simulink model "Diff_Amp"  (Simulink 8.9)
settings: Solver=ode15s  StartTime=0.0  StopTime=0.2  MaxStep=0.00002  RelTol=1e-3  EnableMultiTasking=on
libraries: fl_lib x9, nesl_utility x2
settings Model: Creator=subramanian.krishnan  LastModifiedBy=hac
settings OptimizationCC: ExpressionDepthLimit=2147483647  InitFltsAndDblsToZero=on

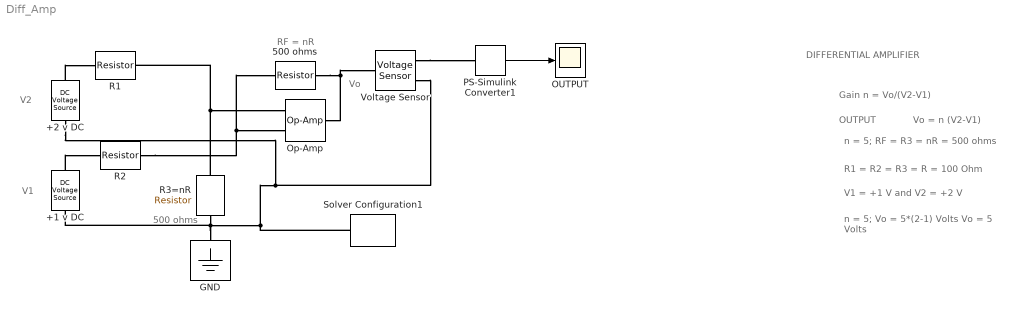
== system Diff_Amp ==
  note: DIFFERENTIAL AMPLIFIER
  note: V2
  note: V1
  note: Vo
  note: Vo = n (V2-V1)
  note: n = 5; Vo = 5*(2-1) Volts
      | Vo = 5 Volts
  note: OUTPUT
  note: RF = nR
  note: R1 = R2 = R3 = R = 100 Ohm
  note: V1 = +1 V and V2 = +2 V
  note: Gain n = Vo/(V2-V1)
  note: 500 ohms
  note: n = 5; RF = R3 = nR = 500 ohms
  +1 v DC : fl_lib/Electrical/Electrical Sources/DC Voltage Source  v0=1 V
  "+2 v DC " : fl_lib/Electrical/Electrical Sources/DC Voltage Source  v0=2 V
  500 ohms : fl_lib/Electrical/Electrical Elements/Resistor  R=500 Ohm  i_specify=off  i_priority=None  i=0 A  i_nominal_specify=off  i_nominal_unit=A  i_nominal_value=1  v_specify=off  v_priority=None  v=0 V  v_nominal_specify=off  v_nominal_unit=V  v_nominal_value=1
  GND : fl_lib/Electrical/Electrical Elements/Electrical Reference
  OUTPUT : Scope
  Op-Amp : fl_lib/Electrical/Electrical Elements/Op-Amp  outI_specify=off  outI_priority=None  outI=0 A  outI_nominal_specify=off  outI_nominal_unit=A  outI_nominal_value=1
  PS-Simulink Converter1 : nesl_utility/PS-Simulink Converter  PhysicalDomain=network_engine_domain  SubClassName=ps_output  LeftPortType=input  RightPortType=output  PseudoPeriodic=off  Frequencies=[]  Unit=1  AffineConversion=off
  R1 : fl_lib/Electrical/Electrical Elements/Resistor  R=100 Ohm  i_specify=off  i_priority=None  i=0 A  i_nominal_specify=off  i_nominal_unit=A  i_nominal_value=1  v_specify=off  v_priority=None  v=0 V  v_nominal_specify=off  v_nominal_unit=V  v_nominal_value=1
  R2 : fl_lib/Electrical/Electrical Elements/Resistor  R=100 Ohm  i_specify=off  i_priority=None  i=0 A  i_nominal_specify=off  i_nominal_unit=A  i_nominal_value=1  v_specify=off  v_priority=None  v=0 V  v_nominal_specify=off  v_nominal_unit=V  v_nominal_value=1
  R3=nR : fl_lib/Electrical/Electrical Elements/Resistor  R=500 Ohm  i_specify=off  i_priority=None  i=0 A  i_nominal_specify=off  i_nominal_unit=A  i_nominal_value=1  v_specify=off  v_priority=None  v=0 V  v_nominal_specify=off  v_nominal_unit=V  v_nominal_value=1
  Solver Configuration1 : nesl_utility/Solver Configuration  PhysicalDomain=network_engine_domain  SubClassName=solver  LeftPortType=input  RightPortType=generic  Accelerate=off  Tones=[]  Harmonics=[]  SimulateNoise=off  Profile=off  UseLocalSampling=off  EnableSwitchedLinearOptims=on  FrequencyDomain=off  UseCCode=off  RelTol=0.001  AbsTol=1e-06  MinStep=1e-09  ToWorkspace=off  RevertToSquareIcSolve=off  NumHomotopyIterations=100  PhasorMode=off  PhasorModeNumHarmonics=1  OverrideAbsTol=off  DoDC=on  ResidualTolerance=1e-9  UseLocalSolver=off  LocalSolverChoice=NE_BACKWARD_EULER_ADVANCER  LocalSolverSampleTime=.001  DoFixedCost=off  MaxNonlinIter=12  MaxModeIter=2  LinearAlgebra=Sparse  DelaysMemoryBudget=1024  AutomaticFiltering=on  FilteringTimeConstant=0.001
  Voltage Sensor : fl_lib/Electrical/Electrical Sensors/Voltage Sensor
  wires:
  PS-Simulink Converter1/1 -> OUTPUT/1
  connections:
  R2/RConn1 -- 500 ohms/LConn1 -- Op-Amp/LConn2
  "+2 v DC "/LConn1 -- R1/LConn1
  +1 v DC/LConn1 -- R2/LConn1
  R3=nR/LConn1 -- R1/RConn1 -- Op-Amp/LConn1
  +1 v DC/RConn1 -- "+2 v DC "/RConn1 -- Voltage Sensor/RConn2 -- Solver Configuration1/RConn1 -- GND/LConn1 -- R3=nR/RConn1
  Op-Amp/RConn1 -- Voltage Sensor/LConn1 -- 500 ohms/RConn1
  Voltage Sensor/RConn1 -- PS-Simulink Converter1/LConn1
